simulink model "Matched_Filter_2"  (R2016b)
settings: Solver=VariableStepAuto  StartTime=0.0  StopTime=10.0  RelTol=1e-3
libraries: commdigbbndam3 x2, commchan3 x1, commsink2 x1, commrandsrc3 x1
settings Model: Creator=ahmed  LastModifiedBy=ahmed

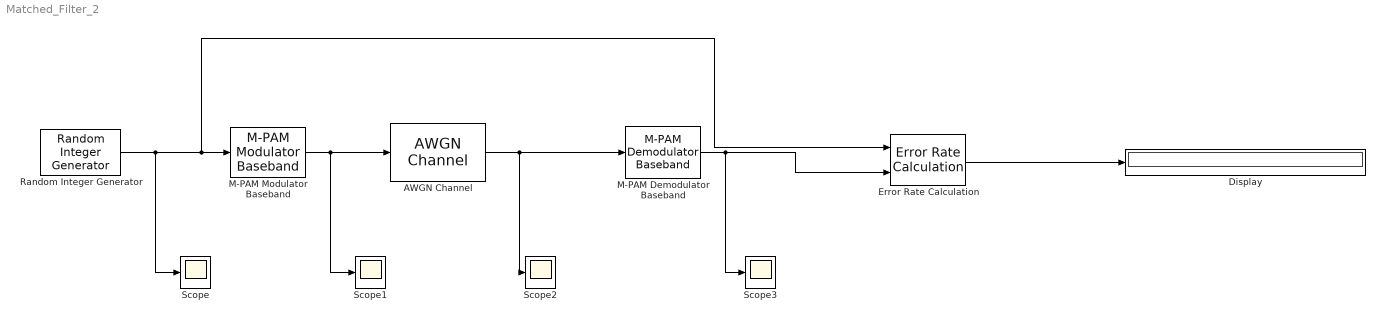
== system Matched_Filter_2 ==
  AWGN Channel : commchan3/AWGN Channel  InputProcessing=Columns as channels (frame based)  seed=15  noiseMode="Signal to noise ratio  (Es/No)"  EbNodB=10  EsNodB=2  SNRdB=10  bitsPerSym=1  Ps=1  Tsym=0.1  variance=1
  Display : Display
  Error Rate Calculation : commsink2/Error Rate Calculation  N=0  st_delay=0  cp_mode=Entire frame  subframe=[]  PMode=Port  WsName=ErrorVec  RsMode2=off  stop=off  numErr=100  maxBits=1e6
  M-PAM Demodulator Baseband : commdigbbndam3/M-PAM Demodulator Baseband  M=8  OutType=Integer  Dec=Binary  PowType=Peak Power  MinDist=2  AvgPow=1  PeakPow=1  outDtype1=Inherit via internal rule  outDtype2=Inherit via internal rule  denormFactorWordLen=16  denormFactorDataTypeStr=Inherit: Same word length as input  denormFactorLastDataTypeStr=Inherit: Same word length as input  prodOutWordLen=16  prodOutRoundingMode=Floor  prodOutOverflowMode=Wrap  prodOutOvFlMode=off  prodOutOvFlModeLastStrValue=off  sumWordLen=16
  M-PAM Modulator Baseband : commdigbbndam3/M-PAM Modulator Baseband  M=8  InType=Integer  Enc=Binary  PowType=Peak Power  MinDist=2  AvgPow=1  PeakPow=1  outDtype=double  outWordLen=16  outUDDataType=sfix(16)  outFracLenMode=Best precision  outFracLen=15  outDataTypeStr=double  outLastDataTypeStr=double
  Random Integer Generator : commrandsrc3/Random Integer Generator  SetSize=8  SeedSource=Parameter  Seed=15  SampleTime=0.1  SamplesPerFrame=1  OutputDataType=double  SimulateUsing=Interpreted execution
  Scope{,1..3} (4 alike) : Scope
  wires:
  M-PAM Modulator Baseband/1 -> Scope1/1, AWGN Channel/1
  AWGN Channel/1 -> Scope2/1, M-PAM Demodulator Baseband/1
  M-PAM Demodulator Baseband/1 -> Scope3/1, Error Rate Calculation/2
  Random Integer Generator/1 -> Scope/1, M-PAM Modulator Baseband/1, Error Rate Calculation/1
  Error Rate Calculation/1 -> Display/1
